simulink model "pto1_gh"  (R2021a)
settings: Solver=VariableStepAuto  StartTime=0.0  StopTime=600  RelTol=1e-3
settings Model: Creator=retou  LastModifiedBy=retou

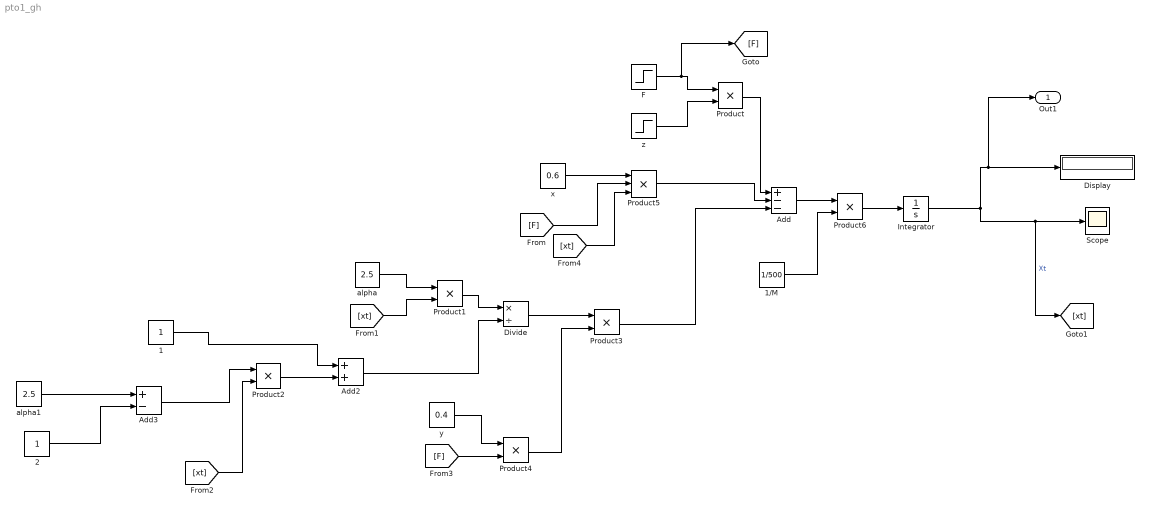
== system pto1_gh ==
  1 : Constant
  1/M : Constant  Value=1/500
  2 : Constant
  Add : Sum  Inputs=+--
  Add2 : Sum
  Add3 : Sum  Inputs=+-
  Display : Display
  Divide : Product  Inputs=*/
  F : Step  Time=0  Before=10  After=10  SampleTime=0
  Integrator : Integrator  InitialCondition=0.410132
  Product{,1..4,6} (6 alike) : Product
  Product5 : Product  Inputs=3
  Scope : Scope
  alpha : Constant  Value=2.5
  alpha1 : Constant  Value=2.5
  x : Constant  Value=0.6
  y : Constant  Value=0.4
  z : Step  Time=0  Before=0.5  After=0.7  SampleTime=0
  Out1 : Outport
  wires:
  F/1 -> [F], Product/1
  z/1 -> Product/2
  Product/1 -> Add/1
  Integrator/1 -> Out1/1, Display/1, [xt], Scope/1  "Xt"
  1/1 -> Add2/1
  alpha1/1 -> Add3/1
  2/1 -> Add3/2
  Add3/1 -> Product2/1
  [xt] -> Product2/2
  Product2/1 -> Add2/2
  [xt] -> Product1/2
  alpha/1 -> Product1/1
  Product1/1 -> Divide/1
  Add2/1 -> Divide/2
  Divide/1 -> Product3/1
  [F] -> Product4/2
  y/1 -> Product4/1
  Product4/1 -> Product3/2
  x/1 -> Product5/1
  [F] -> Product5/2
  Product5/1 -> Add/2
  Product3/1 -> Add/3
  Add/1 -> Product6/1
  1/M/1 -> Product6/2
  Product6/1 -> Integrator/1
  [xt] -> Product5/3
